simulink model "MAE272_HW2_Q1"  (R2023a)
settings: Solver=VariableStepAuto  StartTime=0.0  StopTime=10.0  RelTol=1e-3
model workspace (MAT data in the model file):
  K = 1
values from neighbouring files (symbols this model uses):
  b = 1    [MAE272_hw2_q1.m]
  k = 1    [MAE272_hw2_q1.m]
  m = 1    [MAE272_hw2_q1.m]    (also in fundamental_subspaces.m = size(A, 1))
  M = 2    [MAE272_hw2_q1.m]
settings Model: Creator=kaleb  LastModifiedBy=kaleb

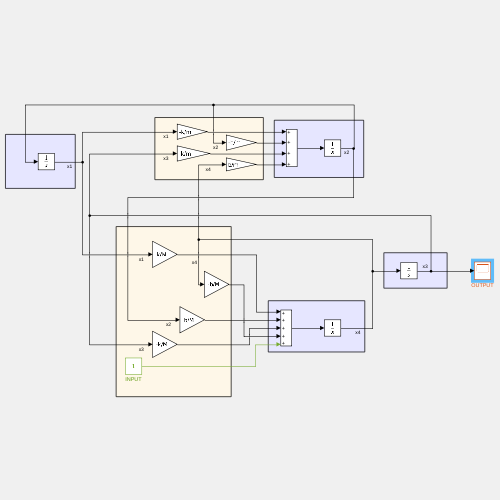
[thumbnail: Simulink's stored preview of the top-level diagram]
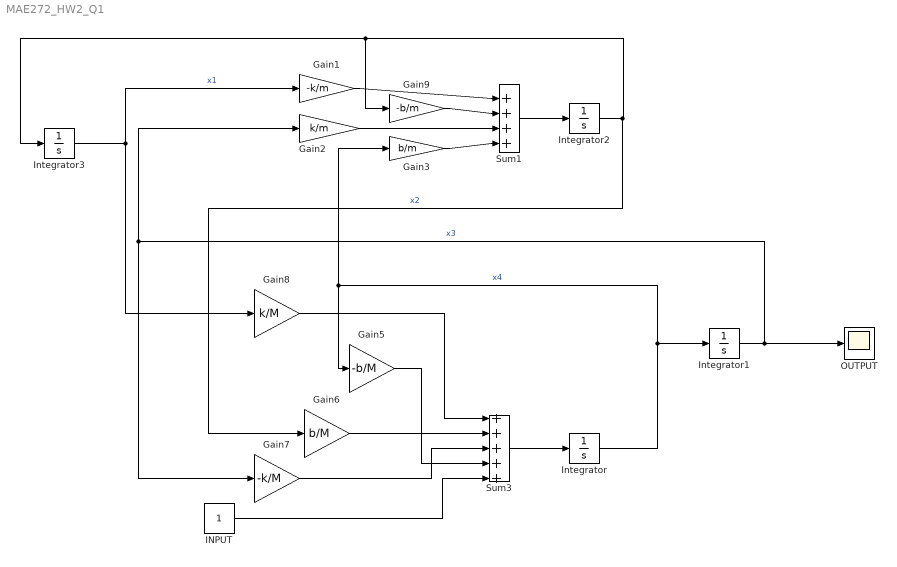
== system MAE272_HW2_Q1 ==
  Gain1 : Gain  Gain=-k/m
  Gain2 : Gain  Gain=k/m
  Gain3 : Gain  Gain=b/m
  Gain5 : Gain  Gain=-b/M
  Gain6 : Gain  Gain=b/M
  Gain7 : Gain  Gain=-k/M
  Gain8 : Gain  Gain=k/M
  Gain9 : Gain  Gain=-b/m
  INPUT : Constant
  Integrator{,1..3} (4 alike) : Integrator
  OUTPUT : Scope
  Sum1 : Sum  Inputs=+|+|+|+
  Sum3 : Sum  Inputs=+++++
  wires:
  Integrator/1 -> Gain3/1, Gain5/1, Integrator1/1  "x4"
  Sum3/1 -> Integrator/1
  Integrator1/1 -> Gain2/1, Gain7/1, OUTPUT/1  "x3"
  Gain7/1 -> Sum3/3
  Gain6/1 -> Sum3/2
  Gain8/1 -> Sum3/1
  Gain5/1 -> Sum3/4
  INPUT/1 -> Sum3/5
  Sum1/1 -> Integrator2/1
  Gain9/1 -> Sum1/2
  Integrator3/1 -> Gain1/1, Gain8/1  "x1"
  Gain1/1 -> Sum1/1
  Gain2/1 -> Sum1/3
  Gain3/1 -> Sum1/4
  Integrator2/1 -> Gain6/1, Integrator3/1, Gain9/1  "x2"
